simulink model "preLab3"  (R2021a)
settings: Solver=VariableStepAuto  StartTime=0.0  StopTime=10  RelTol=1e-3
settings Model: Creator=iumrikhin  LastModifiedBy=iumrikhin

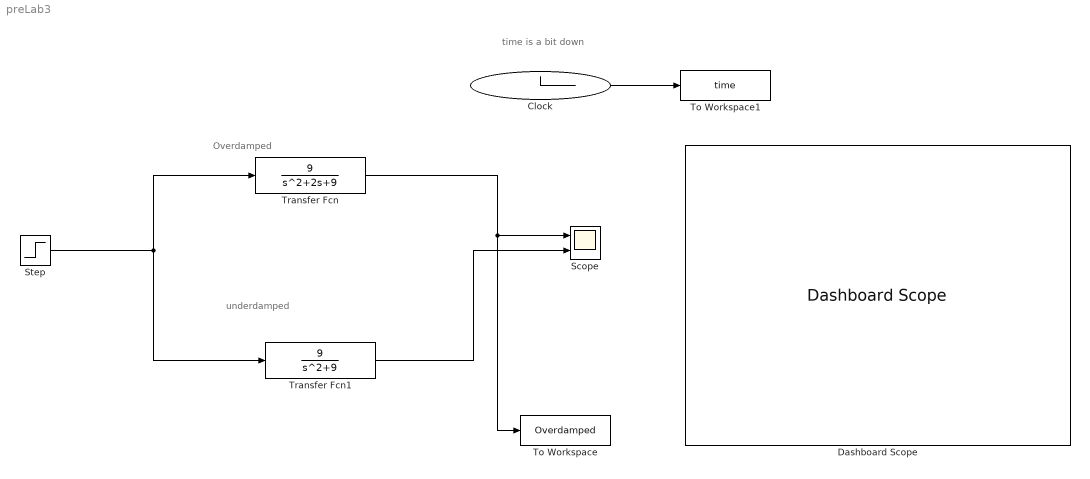
== system preLab3 ==
  note: time is a bit down
  note: Overdamped
  note: underdamped
  Clock : Clock
  Dashboard Scope : DashboardScope
  Scope : Scope  NumInputPorts=2
  Step : Step  SampleTime=0
  To Workspace : ToWorkspace  VariableName=Overdamped  SaveFormat=Timeseries  SampleTime=-1
  To Workspace1 : ToWorkspace  VariableName=time  SaveFormat=Timeseries  SampleTime=-1
  Transfer Fcn : TransferFcn  Numerator=[9]  Denominator=[1 2 9]
  Transfer Fcn1 : TransferFcn  Numerator=[9]  Denominator=[1 0 9]
  wires:
  Transfer Fcn1/1 -> Scope/2
  Transfer Fcn/1 -> Scope/1, To Workspace/1
  Clock/1 -> To Workspace1/1
  Step/1 -> Transfer Fcn/1, Transfer Fcn1/1
